simulink model "raspberrypi_multicore_simple"  (R2021b)
settings: Solver=FixedStepAuto  StartTime=0.0  StopTime=10.0  RelTol=1e-3  EnableMultiTasking=on
undefined symbols (not defined in the file): Green, led0
libraries: simulink x1, raspberrypiBasiclib x1
settings Model: Creator=The MathWorks, Inc.  LastModifiedBy=The MathWorks, Inc.
settings SolverCC: AlgebraicLoopSolver=TrustRegion  PositivePriorityOrder=on
settings OptimizationCC: EnhancedBackFolding=on  PassReuseOutputArgsAs=Individual arguments  ZeroExternalMemoryAtStartup=off  ZeroInternalMemoryAtStartup=off  MaxStackSize=64  OptimizeBlockOrder=speed  DifferentSizesBufferReuse=on  OptimizationCustomize=off  EfficientTunableParamExpr=on
settings DebuggingCC: ParameterTunabilityLossMsg=error  SFMachineParentedDataDiag=warning
settings HardwareCC: ProdBitPerPointer=32  ProdBitPerSizeT=32  ProdBitPerPtrDiffT=32  ProdLargestAtomicInteger=Long  ProdLargestAtomicFloat=Double  ProdWordSize=32  ProdLongLongMode=on  ProdHWDeviceType=ARM Compatible->ARM Cortex
settings RTWCC: Description=Embedded Coder  SystemTargetFile=ert.tlc  HardwareBoard=Raspberry Pi  TLCOptions="-aInlineSetEventsForThisBaseRateFcn=TLC_FALSE -aSuppressMultiTaskScheduler=TLC_FALSE  -aRateBasedStepFcn=0"  TemplateMakefile=ert_default_tmf  Toolchain=GNU GCC Embedded Linux  BuildConfiguration=Faster Runs
settings CodeAppCC: ForceParamTrailComments=on  IgnoreCustomStorageClasses=off  OperatorAnnotations=on  SimulinkDataObjDesc=on  SFDataObjDesc=on  InsertBlockDesc=on
settings ERTTargetCC: SupportVariableSizeSignals=on

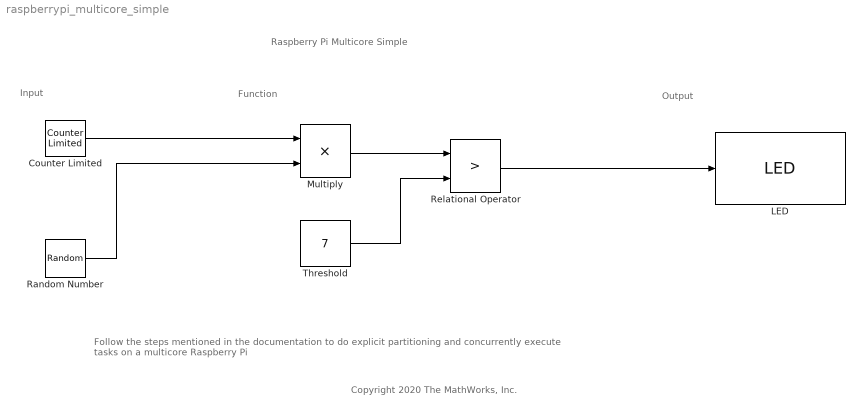
== system raspberrypi_multicore_simple ==
  note: Input
  note: Function
  note: Output
  note: Raspberry Pi Multicore Simple
  note: Copyright 2020 The MathWorks, Inc.
  note: Follow the steps mentioned in the documentation to do explicit partitioning and concurrently execute tasks on a multicore Raspberry Pi
  Counter Limited : simulink/Sources/Counter Limited  uplimit=10  tsamp=0.5
  LED : raspberrypiBasiclib/LED  BoardProperty=Model B Rev2  LED_=led0 (Green)
      settings: SourceProductBaseCode=RASPPI
  Multiply : Product  Inputs=**
  Random Number : RandomNumber  SampleTime=0.5
  Relational Operator : RelationalOperator  Operator=>  OutDataTypeStr=boolean  RndMeth=Nearest
  "Threshold " : Constant  Value=7  OutDataTypeStr=uint8  SampleTime=-1
  wires:
  Random Number/1 -> Multiply/2
  Counter Limited/1 -> Multiply/1
  "Threshold "/1 -> Relational Operator/2
  Relational Operator/1 -> LED/1
  Multiply/1 -> Relational Operator/1
